simulink model "ex_arm_pcont"  (R2023a)
settings: Solver=FixedStepDiscrete  StartTime=0.0  StopTime=5  FixedStep=h  RelTol=1e-3  EnableMultiTasking=on
values from neighbouring files (symbols this model uses):
  kP = 20    [arm_data.mat]
  ref = 90    [arm_data.mat]
libraries: roller485lib x3
settings Model: ExtModeTrigDuration=2  Creator=kawata  LastModifiedBy=kawata
settings SolverCC: AutoInsertRateTranBlk=on
settings DataIOCC: ReturnWorkspaceOutputs=off
settings OptimizationCC: BlockReduction=off  BufferReuse=off  EnhancedBackFolding=on  PassReuseOutputArgsThreshold=0  MaxStackSize=64  OptimizeBlockOrder=speed  DifferentSizesBufferReuse=on
settings DebuggingCC: ParameterTunabilityLossMsg=error
settings HardwareCC: ProdBitPerInt=16  ProdBitPerPointer=16  ProdBitPerSizeT=16  ProdBitPerPtrDiffT=16  ProdLargestAtomicFloat=None  ProdWordSize=8  ProdHWDeviceType=Atmel->AVR
settings SFSimCC: MATLABDynamicMemAlloc=off
settings RTWCC: Description=Embedded Coder  SystemTargetFile=ert.tlc  HardwareBoard=Arduino Mega 2560  TemplateMakefile=ert_default_tmf  Toolchain=Arduino AVR  BuildConfiguration=Faster Runs
settings CodeAppCC: ForceParamTrailComments=on  OperatorAnnotations=on
settings ERTTargetCC: ERTCustomFileBanners=off  SupportContinuousTime=on  SupportNonInlinedSFcns=on  RemoveResetFunc=off  SupportVariableSizeSignals=on  ModelStepFunctionPrototypeControlCompliant=off  ExtModeTransport=3  ExtModeStaticAlloc=on  ExtModeAutomaticAllocSize=off  ExtModeStaticAllocSize=2048  ExtModeMexFile=ext_xcp  ExtModeIntrfLevel=Level2 - Open

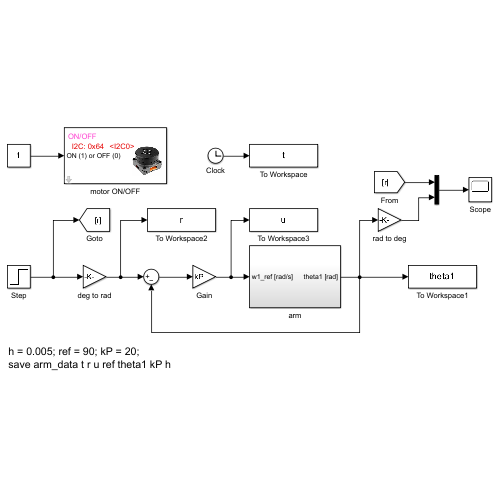
[thumbnail: Simulink's stored preview of the top-level diagram]
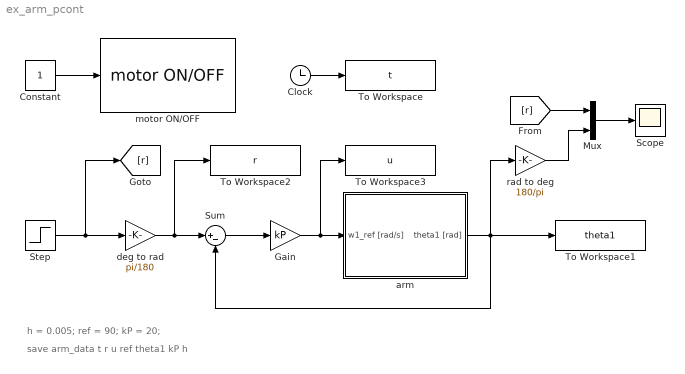
== system ex_arm_pcont ==
  note: h = 0.005; ref = 90; kP = 20;
  note: save arm_data t r u ref theta1 kP h
  Clock : Clock
  Constant : Constant
  Gain : Gain  Gain=kP
  Mux : Mux  Inputs=2
  Scope : Scope
  Step : Step  After=ref  SampleTime=0
  Sum : Sum  Inputs=|+-
  To Workspace : ToWorkspace  VariableName=t  SampleTime=-1
  To Workspace1 : ToWorkspace  VariableName=theta1  SampleTime=-1
  To Workspace2 : ToWorkspace  VariableName=r  SampleTime=-1
  To Workspace3 : ToWorkspace  VariableName=u  SampleTime=-1
  arm : Subsystem
  deg to rad : Gain  Gain=pi/180
  motor ON/OFF : roller485lib/motor ON//OFF  I2CAddress=0x64  I2CModule=0
      settings: SourceProductName=Roller485 Library
  rad to deg : Gain  Gain=180/pi
  wires:
  Gain/1 -> To Workspace3/1, arm/1(w1_ref [rad/s])
  deg to rad/1 -> To Workspace2/1, Sum/1
  Sum/1 -> Gain/1
  Step/1 -> [r], deg to rad/1
  Clock/1 -> To Workspace/1
  arm/1(theta1 [rad]) -> To Workspace1/1, Sum/2, rad to deg/1
  Constant/1 -> motor ON/OFF/1
  Mux/1 -> Scope/1
  [r] -> Mux/1
  rad to deg/1 -> Mux/2

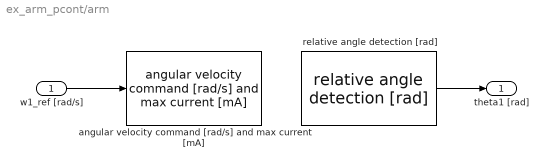
== system ex_arm_pcont/arm ==
  w1_ref [rad/s] : Inport
  angular velocity command [rad/s] and max current [mA] : roller485lib/I2C Write/angular velocity command [rad//s] and max current [mA]  I2CAddress=0x64  I2CModule=0  speed_P=2  speed_I=0  speed_D=850  max_current=1200  set_time1=0  set_time2=0  set_time3=0
      settings: SourceProductName=Roller485 Library
  relative angle detection [rad] : roller485lib/I2C Read/relative angle detection [rad]  I2CAddress=0x64  I2CModule=0  sample_time=-1  set_time=0
      settings: SourceProductName=Roller485 Library
  theta1 [rad] : Outport
  wires:
  w1_ref [rad/s]/1 -> angular velocity command [rad/s] and max current [mA]/1
  relative angle detection [rad]/1 -> theta1 [rad]/1
